simulink model "Snake"  (R2016a)
settings: Solver=VariableStepAuto  StartTime=0.0  StopTime=inf  RelTol=1e-3
libraries: simulink_extras x57, Snake_Lib x44, Arithmetic_Operations_Lib x28, Bit_Multiplexers_Lib x10, Bit_Demultiplexers_Lib x10, commutil2 x6, Decoders_Lib x4, Memory_Blocks_Lib x3, dspsnks4 x1, Miscellaneous x1
(part 1 of 2)
settings Model: Creator=Jozko Mrkvicka  LastModifiedBy=Jozko Mrkvicka

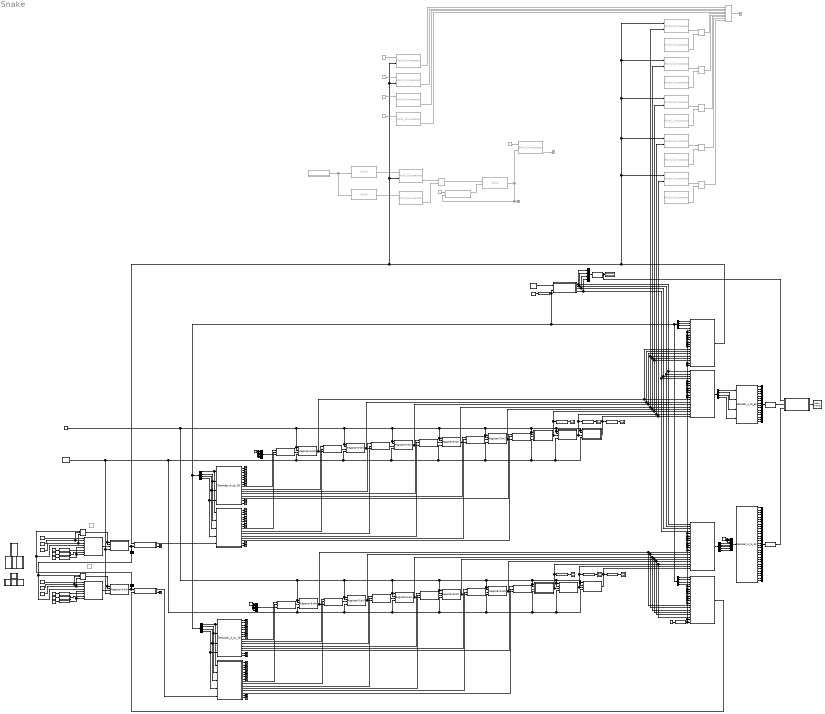
== system Snake ==
  note: New direction is written only when player holds a key.
      | Otherwise old direction keeps latched.
  note: Head is never set to snake position 0 or 1,
  note: TODO:
      |  Add a check to prevent snake from reverting direction. Snake can only turn!!
      | Or figure out how to revert it (idea: maybe it would be possible to shift snake tail directly to it`s head).
  Adder : Subsystem
  Adder1 : Subsystem
  Adder2 : Arithmetic_Operations_Lib/Arithmetic_Operations_Lib/Word_Adder  Commented=on
  Bit to Integer Converter1 : commutil2/Bit to Integer Converter  nbits=32  bitOrder=MSB first  signedOutputValues=Unsigned  outDtype=uint32  outDtypeSigned=Inherit via internal rule
  Bit to Integer Converter2 : commutil2/Bit to Integer Converter  nbits=16  bitOrder=MSB first  signedOutputValues=Unsigned  outDtype=uint32  outDtypeSigned=Inherit via internal rule
  Bit to Integer Converter3 : commutil2/Bit to Integer Converter  nbits=4  bitOrder=MSB first  signedOutputValues=Unsigned  outDtype=uint32  outDtypeSigned=Inherit via internal rule
  Bottom wall : Constant  Commented=on  Value=-1  OutDataTypeStr=boolean
  Bus Creator1 : BusCreator  Inputs=5
  Bus Creator2 : BusCreator  Inputs=5
  Bus Selector : BusSelector  OutputSignals=signal1,signal2,signal3,signal4,signal5
  Bus Selector1 : BusSelector  OutputSignals=signal2,signal3,signal4,signal5
  Bus Selector15 : BusSelector  OutputSignals=signal5
  Bus Selector2 : BusSelector  OutputSignals=signal13,signal14,signal15,signal16
  Bus Selector3 : BusSelector  OutputSignals=signal13,signal14,signal15,signal16
  Bus Selector4 : BusSelector  OutputSignals=signal5
  BusScope(5-bit){,1..5} (6 alike) : Snake_Lib/BusScope(5-bit)
  Counter_4bit : Subsystem
  Decoder_4_to_1 : Decoders_Lib/Decoders_Lib/Decoder_4_to_16
  Decoder_4_to_16 : Decoders_Lib/Decoders_Lib/Decoder_4_to_16
  Decoder_4_to_2 : Decoders_Lib/Decoders_Lib/Decoder_4_to_16
  Decoder_5_to_32 : Decoders_Lib/Decoders_Lib/Decoder_5_to_32
  Delay : Delay  Commented=on  DelayLength=1  InitialCondition=0
  Delay1 : Delay  Commented=on  DelayLength=1  InitialCondition=0
  Demultiplexer_1_to_16(5-bit) : Subsystem  AncestorBlock=Snake_Lib/Demultiplexer_1_to_16(5-bit)
  Demultiplexer_1_to_16(5-bit)1 : Subsystem  AncestorBlock=Snake_Lib/Demultiplexer_1_to_16(5-bit)
  Display{,1..6} (7 alike) : Display
  DisplayClock : simulink_extras/Flip Flops/Clock  period=1
  Down : Constant  Value=0  OutDataTypeStr=boolean
  Game over : Logic  Commented=on  Operator=OR  Inputs=9  IconShape=distinctive  AllPortsSameDT=off  OutDataTypeStr=boolean
  Game over :-( : Terminator  Commented=on
  GameClock : simulink_extras/Flip Flops/Clock  period=6
  General_Purpose_Register_16 (Length of snake) : Memory_Blocks_Lib/Memory_Blocks_Lib/Word  Commented=on
  General_Purpose_Register_16 (Point_to_take(X)) : Memory_Blocks_Lib/Memory_Blocks_Lib/Word  Commented=on
  General_Purpose_Register_16 (Point_to_take(Y)) : Memory_Blocks_Lib/Memory_Blocks_Lib/Word  Commented=on
  Instruction_CMP (Check if snake hit a wall){,,,} (4 alike) : Arithmetic_Operations_Lib/Arithmetic_Operations_Lib/Word_Comparator  Commented=on
  Instruction_CMP (Compare that snake`s head reached new point to take) : Arithmetic_Operations_Lib/Arithmetic_Operations_Lib/Word_Comparator  Commented=on
  Instruction_CMP (Compare that snake`s head reached new point to take) : Arithmetic_Operations_Lib/Arithmetic_Operations_Lib/Word_Comparator  Commented=on
  Instruction_CMP (Check if snake has hit himself){,,1,1..2,2..3,3..4,4} (10 alike) : Arithmetic_Operations_Lib/Arithmetic_Operations_Lib/Word_Comparator  Commented=on
  Instruction_CMP (Check if snake has reached maximal length) : Arithmetic_Operations_Lib/Arithmetic_Operations_Lib/Word_Comparator  Commented=on
  Left : Constant  Value=0  OutDataTypeStr=boolean
  Left wall : Constant  Commented=on  Value=-1  OutDataTypeStr=boolean
  Linear_Feedback_Shift_Register_15bit (random number generator) : Subsystem  Commented=on
  Logical Operator{1..5,9} (6 alike) : Logic  Commented=on  IconShape=distinctive  AllPortsSameDT=off  OutDataTypeStr=boolean
  Logical Operator6 : Logic  Operator=OR  Inputs=3  IconShape=distinctive  AllPortsSameDT=off  OutDataTypeStr=boolean
  Logical Operator7 : Logic  Operator=OR  Inputs=3  IconShape=distinctive  AllPortsSameDT=off  OutDataTypeStr=boolean
  MATLAB Function : MATLAB Function  TreatAsAtomicUnit=on
  Matrix Viewer1 : dspsnks4/Matrix Viewer  ImageParams=off  CMapStr=[0 0.3 0; 0 1 0]  AxisColorbar=on  AxisParams=off  AxisOrigin=Upper left corner  AxisTickMode=Auto  XTickRange=[0 1]  YTickRange=[0 1]  XLabel=X-axis  YLabel=Y-axis  ZLabel=Z-axis  FigPos=[1761 809 160 240]  AxisZoom=on
      settings: YMin=0  YMax=1
  Max length : Constant  Commented=on  Value=16  OutDataTypeStr=boolean
  Multiplexer_2_to_1(5-bit){,1..11} (12 alike) : Snake_Lib/Multiplexer_2_to_1(5-bit)
  Multiplexer_4_to_1_DirSel(5-bit) : Snake_Lib/Multiplexer_4_to_1_DirSel(5-bit)
  Multiplexer_4_to_1_DirSel(5-bit)1 : Snake_Lib/Multiplexer_4_to_1_DirSel(5-bit)
  Mux : Mux  Inputs=16
  Mux1 : Mux  Inputs=32
  Mux2 : Mux  Inputs=8
  Mux3 : Mux
  None1 : Constant  Value=0  OutDataTypeStr=boolean
  None3 : Constant  Value=0  OutDataTypeStr=boolean
  Push Button : Subsystem  DialogController=hmiCreateDDGDialog  IsWebBlock=on  mask(MWDashboardBlock){webBlockId=56926f07-5c30-4489-8789-9949c718d414, webBlockType=pushbutton, ShowInLibBrwoser=on, ShowInitialText=on, HMISrcModelName=Snake}
      mask prompts: webBlockId "WebBlock Id"; webBlockType "WebBlock Type"; HMISrcModelName "Source Model"
      mask Help: helpview([docroot '/mapfiles/simulink.map'], 'hmi_push_button')
      mask Display:
      | model = bdroot(gcb);
      | if strcmp(get_param(model,'BlockDiagramType'), 'library')
      |     image([(matlabroot) '/toolbox/simulink/hmi/icons/PushButton.png']);
      | end
  Push Button1 : Subsystem  DialogController=hmiCreateDDGDialog  IsWebBlock=on  mask(MWDashboardBlock){webBlockId=75882201-b457-4fd9-b9c2-035fbf608d85, webBlockType=pushbutton, ShowInLibBrwoser=on, ShowInitialText=on, HMISrcModelName=Snake}
      mask prompts: webBlockId "WebBlock Id"; webBlockType "WebBlock Type"; HMISrcModelName "Source Model"
      mask Help: helpview([docroot '/mapfiles/simulink.map'], 'hmi_push_button')
      mask Display:
      | model = bdroot(gcb);
      | if strcmp(get_param(model,'BlockDiagramType'), 'library')
      |     image([(matlabroot) '/toolbox/simulink/hmi/icons/PushButton.png']);
      | end
  Push Button2 : Subsystem  DialogController=hmiCreateDDGDialog  IsWebBlock=on  mask(MWDashboardBlock){webBlockId=5ce12bab-ed7e-4f72-890a-6ff3196eb95e, webBlockType=pushbutton, ShowInLibBrwoser=on, ShowInitialText=on, HMISrcModelName=Snake}
      mask prompts: webBlockId "WebBlock Id"; webBlockType "WebBlock Type"; HMISrcModelName "Source Model"
      mask Help: helpview([docroot '/mapfiles/simulink.map'], 'hmi_push_button')
      mask Display:
      | model = bdroot(gcb);
      | if strcmp(get_param(model,'BlockDiagramType'), 'library')
      |     image([(matlabroot) '/toolbox/simulink/hmi/icons/PushButton.png']);
      | end
  Push Button3 : Subsystem  DialogController=hmiCreateDDGDialog  IsWebBlock=on  mask(MWDashboardBlock){webBlockId=28c09741-da14-4d8c-8d5e-be08630d781a, webBlockType=pushbutton, ShowInLibBrwoser=on, ShowInitialText=on, HMISrcModelName=Snake}
      mask prompts: webBlockId "WebBlock Id"; webBlockType "WebBlock Type"; HMISrcModelName "Source Model"
      mask Help: helpview([docroot '/mapfiles/simulink.map'], 'hmi_push_button')
      mask Display:
      | model = bdroot(gcb);
      | if strcmp(get_param(model,'BlockDiagramType'), 'library')
      |     image([(matlabroot) '/toolbox/simulink/hmi/icons/PushButton.png']);
      | end
  Right : Constant  OutDataTypeStr=boolean
  Right wall : Constant  Commented=on  Value=24  OutDataTypeStr=boolean
  Select_Snake_Head(X) : Snake_Lib/Multiplexer_16_to_1(5-bit)
      link override Bus Selector7: OutputSignals=signal1,signal2,signal3,signal4,signal5
  Select_Snake_Head(Y) : Snake_Lib/Multiplexer_16_to_1(5-bit)
      link override Bus Selector7: OutputSignals=signal1,signal2,signal3,signal4,signal5
  Snake Head Position (X) : BusSelector  OutputSignals=signal13,signal14,signal15,signal16
  Snake Head Position (Y) : BusSelector  OutputSignals=signal13,signal14,signal15,signal16
  Snake_X : Snake_Lib/Multiplexer_16_to_1(5-bit)
      link override Bus Selector7: OutputSignals=signal1,signal2,signal3,signal4,signal5
  Snake_X0 : Subsystem
  Snake_X1 : Subsystem
  Snake_X2 : Subsystem
  Snake_X{3..7} (5 alike) : Snake_Lib/Register(5-bit)
  Snake_Y : Snake_Lib/Multiplexer_16_to_1(5-bit)
      link override Bus Creator1: Inputs=5
  Snake_Y0 : Subsystem
  Snake_Y1 : Subsystem
  Snake_Y2 : Subsystem
  Snake_Y{3..7} (5 alike) : Snake_Lib/Register(5-bit)
  Terminator : Terminator  Commented=on
  Terminator{1..3,5..12,20..38,40..51} (42 alike) : Terminator
  Toggle Switch : Subsystem  DialogController=hmiCreateDDGDialog  IsWebBlock=on  mask(MWDashboardBlock){webBlockId=54927be4-b863-4cd1-a632-014d1949c9b6, webBlockType=toggleswitch, ShowInLibBrowser=on, ShowInitialText=on, HMISrcModelName=Snake}
      mask prompts: webBlockId "WebBlock Id"; webBlockType "WebBlock Type"; HMISrcModelName "Source Model"
      mask Help: helpview([docroot '/mapfiles/simulink.map'], 'hmi_toggle_switch')
      mask Display:
      | if strcmp(get_param(bdroot(gcb),'BlockDiagramType'), 'library')
      |     image([(matlabroot) '/toolbox/simulink/hmi/icons/ToggleSwitch.png']);
      | end
  Toggle Switch1 : Subsystem  DialogController=hmiCreateDDGDialog  IsWebBlock=on  mask(MWDashboardBlock){webBlockId=3e42cfe8-21e1-4190-88ba-1de34cedee39, webBlockType=toggleswitch, ShowInLibBrowser=on, ShowInitialText=on, HMISrcModelName=Snake}
      mask prompts: webBlockId "WebBlock Id"; webBlockType "WebBlock Type"; HMISrcModelName "Source Model"
      mask Help: helpview([docroot '/mapfiles/simulink.map'], 'hmi_toggle_switch')
      mask Display:
      | if strcmp(get_param(bdroot(gcb),'BlockDiagramType'), 'library')
      |     image([(matlabroot) '/toolbox/simulink/hmi/icons/ToggleSwitch.png']);
      | end
  Toggle Switch2 : Subsystem  DialogController=hmiCreateDDGDialog  IsWebBlock=on  mask(MWDashboardBlock){webBlockId=c61dffc0-3ed1-4f53-9cab-e3b11f3a47d7, webBlockType=toggleswitch, ShowInLibBrowser=on, ShowInitialText=on, HMISrcModelName=Snake}
      mask prompts: webBlockId "WebBlock Id"; webBlockType "WebBlock Type"; HMISrcModelName "Source Model"
      mask Help: helpview([docroot '/mapfiles/simulink.map'], 'hmi_toggle_switch')
      mask Display:
      | if strcmp(get_param(bdroot(gcb),'BlockDiagramType'), 'library')
      |     image([(matlabroot) '/toolbox/simulink/hmi/icons/ToggleSwitch.png']);
      | end
  Toggle Switch3 : Subsystem  DialogController=hmiCreateDDGDialog  IsWebBlock=on  mask(MWDashboardBlock){webBlockId=f29dcd5f-f5a7-4438-a1c1-2f4b185334c4, webBlockType=toggleswitch, ShowInLibBrowser=on, ShowInitialText=on, HMISrcModelName=Snake}
      mask prompts: webBlockId "WebBlock Id"; webBlockType "WebBlock Type"; HMISrcModelName "Source Model"
      mask Help: helpview([docroot '/mapfiles/simulink.map'], 'hmi_toggle_switch')
      mask Display:
      | if strcmp(get_param(bdroot(gcb),'BlockDiagramType'), 'library')
      |     image([(matlabroot) '/toolbox/simulink/hmi/icons/ToggleSwitch.png']);
      | end
  Top wall : Constant  Commented=on  Value=32  OutDataTypeStr=boolean
  Up : Constant  Value=0  OutDataTypeStr=boolean
  Up1 : Constant  Value=+1  OutDataTypeStr=uint32
  Up2 : Constant  Value=-1  OutDataTypeStr=int8
  Up3 : Constant  Commented=on  Value=+1  OutDataTypeStr=boolean
  Up4 : Constant  Value=+1  OutDataTypeStr=uint32
  Up5 : Constant  Value=-1  OutDataTypeStr=int8
  Up6 : Constant  Value=0  OutDataTypeStr=uint32
  Up7 : Constant  Value=0  OutDataTypeStr=uint32
  Victory!! : Terminator  Commented=on
  X-direction of snake : Subsystem
  Y-direction of snake : Snake_Lib/Register(5-bit)
  const2 : Constant  Value=2  OutDataTypeStr=uint16
  const3 : Constant  OutDataTypeStr=boolean
  const4 : Constant  Value=0  OutDataTypeStr=boolean
  const7 : Constant  Value=0  OutDataTypeStr=boolean
  const8 : Constant  Value=0  OutDataTypeStr=uint8
  const9 : Constant  Value=0  OutDataTypeStr=boolean
  uint_to_bus : Miscellaneous/uint_to_bus
  uint_to_bus(byte){,2..3,5,17} (5 alike) : Snake_Lib/uint_to_bus(byte)
  uint_to_bus(byte)1 : Subsystem
  uint_to_bus(byte)4 : Subsystem
  wires:
  DisplayClock/1 -> Counter_4bit/1(Clock)
  Select_Snake_Head(X)/1 -> Adder/1(Data_In_A(5b)), Instruction_CMP (Check if snake hit a wall)/2, Instruction_CMP (Check if snake hit a wall)/2, Instruction_CMP (Compare that snake`s head reached new point to take)/2, Instruction_CMP (Check if snake has hit himself)4/1, Instruction_CMP (Check if snake has hit himself)3/1, Instruction_CMP (Check if snake has hit himself)2/1, Instruction_CMP (Check if snake has hit himself)1/1, Instruction_CMP (Check if snake has hit himself)/1
  Counter_4bit/2(Addr_2(1b)) -> Mux3/2, Snake_X/2, Snake_Y/2
  Counter_4bit/1(Addr_3(1b)) -> Mux3/1, Snake_X/1, Snake_Y/1
  Counter_4bit/4(Addr_0(1b)) -> Mux3/4, Snake_X/4, Snake_Y/4
  Counter_4bit/3(Addr_1(1b)) -> Mux3/3, Snake_X/3, Snake_Y/3
  Bus Selector1/1 -> Decoder_4_to_16/1  "<signal2>"
  Snake_Y/1 -> Bus Selector/1
  uint_to_bus(byte)/1 -> Multiplexer_4_to_1_DirSel(5-bit)/6
  Multiplexer_4_to_1_DirSel(5-bit)/1 -> X-direction of snake/3(Data(5b))
  uint_to_bus(byte)1/1(Out(5b)) -> Multiplexer_4_to_1_DirSel(5-bit)/7
  Right/1 -> Logical Operator6/2, Multiplexer_4_to_1_DirSel(5-bit)/2
  Left/1 -> Logical Operator6/3, Multiplexer_4_to_1_DirSel(5-bit)/3
  General_Purpose_Register_16 (Point_to_take(X))/1 -> Instruction_CMP (Compare that snake`s head reached new point to take)/1
  Linear_Feedback_Shift_Register_15bit (random number generator)/1(Random_Number(2B)) -> General_Purpose_Register_16 (Point_to_take(Y))/3, General_Purpose_Register_16 (Point_to_take(X))/3
  General_Purpose_Register_16 (Length of snake)/1 -> Terminator/1, Adder2/2, Instruction_CMP (Check if snake has reached maximal length)/2
  Up3/1 -> Adder2/1
  Instruction_CMP (Compare that snake`s head reached new point to take)/5 -> Logical Operator9/1
  Logical Operator9/1 -> General_Purpose_Register_16 (Length of snake)/2
  General_Purpose_Register_16 (Point_to_take(Y))/1 -> Instruction_CMP (Compare that snake`s head reached new point to take)/1
  Instruction_CMP (Compare that snake`s head reached new point to take)/5 -> Logical Operator9/2
  Adder2/1 -> General_Purpose_Register_16 (Length of snake)/3
  Left wall/1 -> Instruction_CMP (Check if snake hit a wall)/1
  Instruction_CMP (Check if snake hit a wall)/5 -> Game over/2
  Right wall/1 -> Instruction_CMP (Check if snake hit a wall)/1
  Instruction_CMP (Check if snake hit a wall)/5 -> Game over/1
  Bottom wall/1 -> Instruction_CMP (Check if snake hit a wall)/1
  Top wall/1 -> Instruction_CMP (Check if snake hit a wall)/1
  Instruction_CMP (Check if snake hit a wall)/5 -> Game over/4
  Instruction_CMP (Check if snake hit a wall)/5 -> Game over/3
  Max length/1 -> Instruction_CMP (Check if snake has reached maximal length)/1
  Instruction_CMP (Check if snake has reached maximal length)/5 -> Victory!!/1
  Game over/1 -> Game over :-(/1
  Instruction_CMP (Check if snake has hit himself)/5 -> Logical Operator1/1
  Instruction_CMP (Check if snake has hit himself)/5 -> Logical Operator1/2
  Logical Operator1/1 -> Game over/5
  Instruction_CMP (Check if snake has hit himself)1/5 -> Logical Operator2/1
  Instruction_CMP (Check if snake has hit himself)1/5 -> Logical Operator2/2
  Instruction_CMP (Check if snake has hit himself)2/5 -> Logical Operator3/1
  Instruction_CMP (Check if snake has hit himself)2/5 -> Logical Operator3/2
  Instruction_CMP (Check if snake has hit himself)3/5 -> Logical Operator4/1
  Instruction_CMP (Check if snake has hit himself)3/5 -> Logical Operator4/2
  Instruction_CMP (Check if snake has hit himself)4/5 -> Logical Operator5/1
  Instruction_CMP (Check if snake has hit himself)4/5 -> Logical Operator5/2
  Logical Operator2/1 -> Game over/6
  Logical Operator3/1 -> Game over/7
  Logical Operator4/1 -> Game over/8
  Logical Operator5/1 -> Game over/9
  Decoder_4_to_16/1 -> Mux/1
  Decoder_4_to_16/2 -> Mux/2
  Decoder_4_to_16/3 -> Mux/3
  Decoder_4_to_16/4 -> Mux/4
  Decoder_4_to_16/5 -> Mux/5
  Decoder_4_to_16/6 -> Mux/6
  Decoder_4_to_16/7 -> Mux/7
  Decoder_4_to_16/8 -> Mux/8
  Decoder_4_to_16/9 -> Mux/9
  Decoder_4_to_16/10 -> Mux/10
  Decoder_4_to_16/11 -> Mux/11
  Decoder_4_to_16/12 -> Mux/12
  Decoder_4_to_16/13 -> Mux/13
  Decoder_4_to_16/14 -> Mux/14
  Decoder_4_to_16/15 -> Mux/15
  Decoder_4_to_16/16 -> Mux/16
  Mux/1 -> Bit to Integer Converter2/1
  Bus Selector1/2 -> Decoder_4_to_16/2  "<signal3>"
  Bus Selector1/3 -> Decoder_4_to_16/3  "<signal4>"
  Bus Selector1/4 -> Decoder_4_to_16/4  "<signal5>"
  Decoder_5_to_32/1 -> Mux1/1
  Decoder_5_to_32/2 -> Mux1/2
  Decoder_5_to_32/3 -> Mux1/3
  Decoder_5_to_32/4 -> Mux1/4
  Decoder_5_to_32/5 -> Mux1/5
  Decoder_5_to_32/6 -> Mux1/6
  Decoder_5_to_32/7 -> Mux1/7
  Decoder_5_to_32/8 -> Mux1/8
  Decoder_5_to_32/9 -> Mux1/9
  Decoder_5_to_32/10 -> Mux1/10
  Decoder_5_to_32/11 -> Mux1/11
  Decoder_5_to_32/12 -> Mux1/12
  Decoder_5_to_32/13 -> Mux1/13
  Decoder_5_to_32/14 -> Mux1/14
  Decoder_5_to_32/15 -> Mux1/15
  Decoder_5_to_32/16 -> Mux1/16
  Decoder_5_to_32/17 -> Mux1/17
  Decoder_5_to_32/18 -> Mux1/18
  Decoder_5_to_32/19 -> Mux1/19
  Decoder_5_to_32/20 -> Mux1/20
  Decoder_5_to_32/21 -> Mux1/21
  Decoder_5_to_32/22 -> Mux1/22
  Decoder_5_to_32/23 -> Mux1/23
  Decoder_5_to_32/24 -> Mux1/24
  Decoder_5_to_32/25 -> Mux1/25
  Decoder_5_to_32/26 -> Mux1/26
  Decoder_5_to_32/27 -> Mux1/27
  Decoder_5_to_32/28 -> Mux1/28
  Decoder_5_to_32/29 -> Mux1/29
  Decoder_5_to_32/30 -> Mux1/30
  Decoder_5_to_32/31 -> Mux1/31
  Mux1/1 -> Bit to Integer Converter1/1
  Decoder_5_to_32/32 -> Mux1/32
  const2/1 -> uint_to_bus/1
  Bus Selector/1 -> Mux2/4  "<signal1>"
  Bus Selector/2 -> Mux2/5  "<signal2>"
  Bus Selector/3 -> Mux2/6  "<signal3>"
  Bus Selector/4 -> Mux2/7  "<signal4>"
  Bus Selector/5 -> Mux2/8  "<signal5>"
  Mux2/1 -> Decoder_5_to_32/1
  const7/1 -> Mux2/2, Mux2/3, Mux2/1
  Snake_X/1 -> Bus Selector1/1
  const9/1 -> Bus Creator1/5, Bus Creator1/4, Bus Creator1/3, Bus Creator1/2, Bus Creator1/1
  Bus Creator1/1 -> Multiplexer_2_to_1(5-bit)/3
  Mux3/1 -> Bit to Integer Converter3/1
  Adder/2(Carry_Out(1b)) -> Terminator1/1
  Adder/1(Data_Out(5b)) -> Demultiplexer_1_to_16(5-bit)/5(Data(5b))
  MATLAB Function/1(Framebuffer) -> Matrix Viewer1/1
  Bit to Integer Converter2/1 -> MATLAB Function/2(x)
  Bit to Integer Converter1/1 -> MATLAB Function/3(y)
  Snake_X7/1 -> Multiplexer_2_to_1(5-bit)1/3, Snake_X/13, Select_Snake_Head(X)/13
  Snake_X6/1 -> Multiplexer_2_to_1(5-bit)2/3, Snake_X/14, Select_Snake_Head(X)/14
  Snake_X5/1 -> Multiplexer_2_to_1(5-bit)3/3, Snake_X/15, Select_Snake_Head(X)/15
  Snake_X4/1 -> Multiplexer_2_to_1(5-bit)4/3, Instruction_CMP (Check if snake has hit himself)/2, Select_Snake_Head(X)/16, Snake_X/16
  Snake_X3/1 -> Multiplexer_2_to_1(5-bit)5/3, Instruction_CMP (Check if snake has hit himself)1/2, Select_Snake_Head(X)/17, Snake_X/17
  Snake_X2/1(DataOut(5b)) -> Snake_X1/3(Data(5b)), Instruction_CMP (Check if snake has hit himself)2/2, Select_Snake_Head(X)/18, Snake_X/18, BusScope(5-bit)1/1
  Snake_X1/1(DataOut(5b)) -> BusScope(5-bit)/1, Snake_X/19, Instruction_CMP (Check if snake has hit himself)3/2, Snake_X0/3(Data(5b))
  Snake_X0/1(DataOut(5b)) -> BusScope(5-bit)2/1, Snake_X/20, Instruction_CMP (Check if snake has hit himself)4/2
  Bit to Integer Converter3/1 -> MATLAB Function/1(cnt), Display/1
  Bus Selector4/1 -> Multiplexer_4_to_1_DirSel(5-bit)/4, Logical Operator6/1  "<signal5>"
  uint_to_bus(byte)2/1 -> Multiplexer_4_to_1_DirSel(5-bit)/8, Multiplexer_4_to_1_DirSel(5-bit)/5
  None1/1 -> Multiplexer_4_to_1_DirSel(5-bit)/1
  Bus Selector2/1 -> Select_Snake_Head(X)/1  "<signal13>"
  Bus Selector2/2 -> Select_Snake_Head(X)/2  "<signal14>"
  Bus Selector2/3 -> Select_Snake_Head(X)/3  "<signal15>"
  Bus Selector2/4 -> Select_Snake_Head(X)/4  "<signal16>"
  const8/1 -> uint_to_bus(byte)17/1
  Snake Head Position (X)/1 -> Decoder_4_to_1/1, Demultiplexer_1_to_16(5-bit)/1(Addr3(1b))  "<signal13>"
  Snake Head Position (X)/2 -> Decoder_4_to_1/2, Demultiplexer_1_to_16(5-bit)/2(Addr2(1b))  "<signal14>"
  Snake Head Position (X)/3 -> Decoder_4_to_1/3, Demultiplexer_1_to_16(5-bit)/3(Addr1(1b))  "<signal15>"
  Snake Head Position (X)/4 -> Decoder_4_to_1/4, Demultiplexer_1_to_16(5-bit)/4(Addr0(1b))  "<signal16>"
  uint_to_bus/1 -> Counter_4bit/2(Snake_Length(2B)), Bus Selector3/1, Bus Selector2/1, Snake Head Position (Y)/1, Snake Head Position (X)/1
  Demultiplexer_1_to_16(5-bit)/15(Data_01(5b)) -> Terminator2/1
  Demultiplexer_1_to_16(5-bit)/16(Data_00(5b)) -> Terminator3/1
  Multiplexer_2_to_1(5-bit)/1 -> Snake_X7/3
  Multiplexer_2_to_1(5-bit)1/1 -> Snake_X6/3
  Multiplexer_2_to_1(5-bit)2/1 -> Snake_X5/3
  Multiplexer_2_to_1(5-bit)3/1 -> Snake_X4/3
  Multiplexer_2_to_1(5-bit)4/1 -> Snake_X3/3
  Multiplexer_2_to_1(5-bit)5/1 -> Snake_X2/3(Data(5b))
  Decoder_4_to_1/9 -> Multiplexer_2_to_1(5-bit)/1
  Demultiplexer_1_to_16(5-bit)/9(Data_07(5b)) -> Multiplexer_2_to_1(5-bit)/2
  Decoder_4_to_1/10 -> Multiplexer_2_to_1(5-bit)1/1
  Demultiplexer_1_to_16(5-bit)/10(Data_06(5b)) -> Multiplexer_2_to_1(5-bit)1/2
  Decoder_4_to_1/11 -> Multiplexer_2_to_1(5-bit)2/1
  Demultiplexer_1_to_16(5-bit)/11(Data_05(5b)) -> Multiplexer_2_to_1(5-bit)2/2
  Decoder_4_to_1/12 -> Multiplexer_2_to_1(5-bit)3/1
  Demultiplexer_1_to_16(5-bit)/12(Data_04(5b)) -> Multiplexer_2_to_1(5-bit)3/2
  Decoder_4_to_1/13 -> Multiplexer_2_to_1(5-bit)4/1
  Demultiplexer_1_to_16(5-bit)/13(Data_03(5b)) -> Multiplexer_2_to_1(5-bit)4/2
  Decoder_4_to_1/14 -> Multiplexer_2_to_1(5-bit)5/1
  Demultiplexer_1_to_16(5-bit)/14(Data_02(5b)) -> Multiplexer_2_to_1(5-bit)5/2
  Demultiplexer_1_to_16(5-bit)/1(Data_15(5b)) -> Terminator20/1
  Demultiplexer_1_to_16(5-bit)/2(Data_14(5b)) -> Terminator21/1
  Demultiplexer_1_to_16(5-bit)/3(Data_13(5b)) -> Terminator22/1
  Demultiplexer_1_to_16(5-bit)/4(Data_12(5b)) -> Terminator23/1
  Demultiplexer_1_to_16(5-bit)/5(Data_11(5b)) -> Terminator24/1
  Demultiplexer_1_to_16(5-bit)/6(Data_10(5b)) -> Terminator25/1
  Demultiplexer_1_to_16(5-bit)/7(Data_09(5b)) -> Terminator26/1
  Demultiplexer_1_to_16(5-bit)/8(Data_08(5b)) -> Terminator27/1
  Decoder_4_to_1/1 -> Terminator28/1
  Decoder_4_to_1/2 -> Terminator29/1
  Decoder_4_to_1/3 -> Terminator30/1
  Decoder_4_to_1/4 -> Terminator31/1
  Decoder_4_to_1/5 -> Terminator32/1
  Decoder_4_to_1/6 -> Terminator33/1
  Decoder_4_to_1/7 -> Terminator34/1
  Decoder_4_to_1/8 -> Terminator35/1
  Decoder_4_to_1/15 -> Terminator36/1
  Decoder_4_to_1/16 -> Terminator37/1
  Up1/1 -> uint_to_bus(byte)/1
  Up2/1 -> uint_to_bus(byte)1/1(In(5b))
  Up6/1 -> uint_to_bus(byte)2/1
  BusScope(5-bit)/1 -> Display2/1
  BusScope(5-bit)1/1 -> Display1/1
  BusScope(5-bit)2/1 -> Display3/1
  GameClock/1 -> Y-direction of snake/4, X-direction of snake/4(CLK), Snake_X0/4(CLK), Snake_X1/4(CLK), Snake_X2/4(CLK), Snake_X3/4, Snake_X4/4, Snake_X5/4, Snake_X6/4, Snake_X7/4, Snake_Y0/4(CLK), Snake_Y1/4(CLK), Snake_Y2/4(CLK), Snake_Y3/4, Snake_Y4/4, Snake_Y5/4, Snake_Y6/4, Snake_Y7/4
  const4/1 -> Bus Creator2/5, Bus Creator2/4, Bus Creator2/3, Bus Creator2/2, Bus Creator2/1
  Bus Creator2/1 -> Multiplexer_2_to_1(5-bit)6/3
  Snake_Y7/1 -> Multiplexer_2_to_1(5-bit)7/3, Snake_Y/13, Select_Snake_Head(Y)/13
  Snake_Y6/1 -> Multiplexer_2_to_1(5-bit)8/3, Snake_Y/14, Select_Snake_Head(Y)/14
  Snake_Y5/1 -> Multiplexer_2_to_1(5-bit)9/3, Snake_Y/15, Select_Snake_Head(Y)/15
  Snake_Y4/1 -> Multiplexer_2_to_1(5-bit)10/3, Snake_Y/16, Select_Snake_Head(Y)/16
  Snake_Y3/1 -> Multiplexer_2_to_1(5-bit)11/3, Snake_Y/17, Select_Snake_Head(Y)/17
  Snake_Y2/1(DataOut(5b)) -> Snake_Y1/3(Data(5b)), Snake_Y/18, Select_Snake_Head(Y)/18, BusScope(5-bit)4/1
  Snake_Y1/1(DataOut(5b)) -> Snake_Y/19, BusScope(5-bit)3/1, Snake_Y0/3(Data(5b))
  Snake_Y0/1(DataOut(5b)) -> Snake_Y/20, BusScope(5-bit)5/1
  Snake Head Position (Y)/1 -> Decoder_4_to_2/1, Demultiplexer_1_to_16(5-bit)1/1(Addr3(1b))  "<signal13>"
  Snake Head Position (Y)/2 -> Decoder_4_to_2/2, Demultiplexer_1_to_16(5-bit)1/2(Addr2(1b))  "<signal14>"
  Snake Head Position (Y)/3 -> Decoder_4_to_2/3, Demultiplexer_1_to_16(5-bit)1/3(Addr1(1b))  "<signal15>"
  Snake Head Position (Y)/4 -> Decoder_4_to_2/4, Demultiplexer_1_to_16(5-bit)1/4(Addr0(1b))  "<signal16>"
  Demultiplexer_1_to_16(5-bit)1/15(Data_01(5b)) -> Terminator5/1
  Demultiplexer_1_to_16(5-bit)1/16(Data_00(5b)) -> Terminator43/1
  Multiplexer_2_to_1(5-bit)6/1 -> Snake_Y7/3
  Multiplexer_2_to_1(5-bit)7/1 -> Snake_Y6/3
  Multiplexer_2_to_1(5-bit)8/1 -> Snake_Y5/3
  Multiplexer_2_to_1(5-bit)9/1 -> Snake_Y4/3
  Multiplexer_2_to_1(5-bit)10/1 -> Snake_Y3/3
  Multiplexer_2_to_1(5-bit)11/1 -> Snake_Y2/3(Data(5b))
  Decoder_4_to_2/9 -> Multiplexer_2_to_1(5-bit)6/1
  Demultiplexer_1_to_16(5-bit)1/9(Data_07(5b)) -> Multiplexer_2_to_1(5-bit)6/2
  Decoder_4_to_2/10 -> Multiplexer_2_to_1(5-bit)7/1
  Demultiplexer_1_to_16(5-bit)1/10(Data_06(5b)) -> Multiplexer_2_to_1(5-bit)7/2
  Decoder_4_to_2/11 -> Multiplexer_2_to_1(5-bit)8/1
  Demultiplexer_1_to_16(5-bit)1/11(Data_05(5b)) -> Multiplexer_2_to_1(5-bit)8/2
  Decoder_4_to_2/12 -> Multiplexer_2_to_1(5-bit)9/1
  Demultiplexer_1_to_16(5-bit)1/12(Data_04(5b)) -> Multiplexer_2_to_1(5-bit)9/2
  Decoder_4_to_2/13 -> Multiplexer_2_to_1(5-bit)10/1
  Demultiplexer_1_to_16(5-bit)1/13(Data_03(5b)) -> Multiplexer_2_to_1(5-bit)10/2
  Decoder_4_to_2/14 -> Multiplexer_2_to_1(5-bit)11/1
  Demultiplexer_1_to_16(5-bit)1/14(Data_02(5b)) -> Multiplexer_2_to_1(5-bit)11/2
  Demultiplexer_1_to_16(5-bit)1/1(Data_15(5b)) -> Terminator6/1
  Demultiplexer_1_to_16(5-bit)1/2(Data_14(5b)) -> Terminator7/1
  Demultiplexer_1_to_16(5-bit)1/3(Data_13(5b)) -> Terminator8/1
  Demultiplexer_1_to_16(5-bit)1/4(Data_12(5b)) -> Terminator9/1
  Demultiplexer_1_to_16(5-bit)1/5(Data_11(5b)) -> Terminator10/1
  Demultiplexer_1_to_16(5-bit)1/6(Data_10(5b)) -> Terminator11/1
  Demultiplexer_1_to_16(5-bit)1/7(Data_09(5b)) -> Terminator12/1
  Demultiplexer_1_to_16(5-bit)1/8(Data_08(5b)) -> Terminator40/1
  Decoder_4_to_2/1 -> Terminator41/1
  Decoder_4_to_2/2 -> Terminator42/1
  Decoder_4_to_2/3 -> Terminator44/1
  Decoder_4_to_2/4 -> Terminator45/1
  Decoder_4_to_2/5 -> Terminator46/1
  Decoder_4_to_2/6 -> Terminator47/1
  Decoder_4_to_2/7 -> Terminator48/1
  Decoder_4_to_2/8 -> Terminator49/1
  Decoder_4_to_2/15 -> Terminator50/1
  Decoder_4_to_2/16 -> Terminator51/1
  BusScope(5-bit)3/1 -> Display5/1
  BusScope(5-bit)4/1 -> Display4/1
  BusScope(5-bit)5/1 -> Display6/1
  Bus Selector3/1 -> Select_Snake_Head(Y)/1  "<signal13>"
  Bus Selector3/2 -> Select_Snake_Head(Y)/2  "<signal14>"
  Bus Selector3/3 -> Select_Snake_Head(Y)/3  "<signal15>"
  Bus Selector3/4 -> Select_Snake_Head(Y)/4  "<signal16>"
  uint_to_bus(byte)17/1 -> Select_Snake_Head(X)/5, Select_Snake_Head(X)/6, Select_Snake_Head(X)/7, Select_Snake_Head(X)/8, Select_Snake_Head(X)/9, Select_Snake_Head(X)/10, Select_Snake_Head(X)/11, Select_Snake_Head(X)/12, Select_Snake_Head(X)/19, Select_Snake_Head(X)/20, Snake_X/5, Snake_X/6, Snake_X/7, Snake_X/8, Snake_X/9, Snake_X/10, Snake_X/11, Snake_X/12, Snake_Y/5, Snake_Y/6, Snake_Y/7, Snake_Y/8, Snake_Y/9, Snake_Y/10, Snake_Y/11, Snake_Y/12, Select_Snake_Head(Y)/5, Select_Snake_Head(Y)/6, Select_Snake_Head(Y)/7, Select_Snake_Head(Y)/8, Select_Snake_Head(Y)/9, Select_Snake_Head(Y)/10, Select_Snake_Head(Y)/11, Select_Snake_Head(Y)/12, Select_Snake_Head(Y)/19, Select_Snake_Head(Y)/20
  uint_to_bus(byte)3/1 -> Multiplexer_4_to_1_DirSel(5-bit)1/6
  Multiplexer_4_to_1_DirSel(5-bit)1/1 -> Y-direction of snake/3
  uint_to_bus(byte)4/1(Out(5b)) -> Multiplexer_4_to_1_DirSel(5-bit)1/7
  Down/1 -> Logical Operator7/2, Multiplexer_4_to_1_DirSel(5-bit)1/2
  Up/1 -> Logical Operator7/3, Multiplexer_4_to_1_DirSel(5-bit)1/3
  Adder1/2(Carry_Out(1b)) -> Terminator38/1
  uint_to_bus(byte)5/1 -> Multiplexer_4_to_1_DirSel(5-bit)1/8, Multiplexer_4_to_1_DirSel(5-bit)1/5
  None3/1 -> Multiplexer_4_to_1_DirSel(5-bit)1/1
  Up4/1 -> uint_to_bus(byte)3/1
  Up5/1 -> uint_to_bus(byte)4/1(In(5b))
  Up7/1 -> uint_to_bus(byte)5/1
  Adder1/1(Data_Out(5b)) -> Demultiplexer_1_to_16(5-bit)1/5(Data(5b))
  Select_Snake_Head(Y)/1 -> Adder1/2(Data_In_B(5b))
  X-direction of snake/1(DataOut(5b)) -> Bus Selector15/1, Adder/2(Data_In_B(5b))
  Y-direction of snake/1 -> Adder1/1(Data_In_A(5b)), Bus Selector4/1
  const3/1 -> Snake_Y0/2(Write(1b)), Snake_Y0/1(Select(1b)), Snake_Y1/1(Select(1b)), Snake_Y1/2(Write(1b)), Snake_Y2/1(Select(1b)), Snake_Y2/2(Write(1b)), Snake_Y3/2, Snake_Y3/1, Snake_Y4/1, Snake_Y4/2, Snake_Y5/1, Snake_Y5/2, Snake_Y6/1, Snake_Y6/2, Snake_Y7/1, Snake_Y7/2, Snake_X0/2(Write(1b)), Snake_X0/1(Select(1b)), Snake_X1/2(Write(1b)), Snake_X1/1(Select(1b)), Snake_X2/1(Select(1b)), Snake_X2/2(Write(1b)), Snake_X3/1, Snake_X3/2, Snake_X4/2, Snake_X4/1, Snake_X5/2, Snake_X5/1, Snake_X6/1, Snake_X6/2, Snake_X7/2, Snake_X7/1
  Logical Operator6/1 -> X-direction of snake/1(Select(1b)), X-direction of snake/2(Write(1b))
  Logical Operator7/1 -> Y-direction of snake/1, Y-direction of snake/2
  Bus Selector15/1 -> Logical Operator7/1, Multiplexer_4_to_1_DirSel(5-bit)1/4  "<signal5>"

== system Snake/Adder ==
  Data_In_A(5b) : Inport
  Data_In_B(5b) : Inport  Port=2
  Bit_Adder_(0) : Arithmetic_Operations_Lib/Arithmetic_Operations_Lib/Bit_Adder
  Bit_Adder_(1) : Arithmetic_Operations_Lib/Arithmetic_Operations_Lib/Bit_Adder
  Bit_Adder_(2) : Arithmetic_Operations_Lib/Arithmetic_Operations_Lib/Bit_Adder
  Bit_Adder_(3) : Arithmetic_Operations_Lib/Arithmetic_Operations_Lib/Bit_Adder
  Bit_Adder_(4) : Arithmetic_Operations_Lib/Arithmetic_Operations_Lib/Bit_Adder
  Bus Creator : BusCreator  Inputs=5
  Bus Selector : BusSelector  OutputSignals=signal1,signal2,signal3,signal4,signal5
  Bus Selector1 : BusSelector  OutputSignals=signal1,signal2,signal3,signal4,signal5
  Constant : Constant  Value=0
  Data_Out(5b) : Outport
  Carry_Out(1b) : Outport  Port=2
  wires:
  Bit_Adder_(4)/2 -> Carry_Out(1b)/1
  Data_In_A(5b)/1 -> Bus Selector/1
  Data_In_B(5b)/1 -> Bus Selector1/1
  Bus Creator/1 -> Data_Out(5b)/1
  Bit_Adder_(0)/1 -> Bus Creator/5
  Bit_Adder_(1)/1 -> Bus Creator/4
  Bit_Adder_(2)/1 -> Bus Creator/3
  Bit_Adder_(4)/1 -> Bus Creator/1
  Bit_Adder_(3)/1 -> Bus Creator/2
  Bus Selector/1 -> Bit_Adder_(4)/1  "<signal1>"
  Bus Selector/2 -> Bit_Adder_(3)/1  "<signal2>"
  Bus Selector/3 -> Bit_Adder_(2)/1  "<signal3>"
  Bus Selector/4 -> Bit_Adder_(1)/1  "<signal4>"
  Bus Selector/5 -> Bit_Adder_(0)/1  "<signal5>"
  Bus Selector1/1 -> Bit_Adder_(4)/2  "<signal1>"
  Bus Selector1/2 -> Bit_Adder_(3)/2  "<signal2>"
  Bus Selector1/3 -> Bit_Adder_(2)/2  "<signal3>"
  Bus Selector1/4 -> Bit_Adder_(1)/2  "<signal4>"
  Bus Selector1/5 -> Bit_Adder_(0)/2  "<signal5>"
  Constant/1 -> Bit_Adder_(0)/3
  Bit_Adder_(0)/2 -> Bit_Adder_(1)/3
  Bit_Adder_(1)/2 -> Bit_Adder_(2)/3
  Bit_Adder_(2)/2 -> Bit_Adder_(3)/3
  Bit_Adder_(3)/2 -> Bit_Adder_(4)/3

== system Snake/Adder1 ==
  Data_In_A(5b) : Inport
  Data_In_B(5b) : Inport  Port=2
  Bit_Adder_(0) : Arithmetic_Operations_Lib/Arithmetic_Operations_Lib/Bit_Adder
  Bit_Adder_(1) : Arithmetic_Operations_Lib/Arithmetic_Operations_Lib/Bit_Adder
  Bit_Adder_(2) : Arithmetic_Operations_Lib/Arithmetic_Operations_Lib/Bit_Adder
  Bit_Adder_(3) : Arithmetic_Operations_Lib/Arithmetic_Operations_Lib/Bit_Adder
  Bit_Adder_(4) : Arithmetic_Operations_Lib/Arithmetic_Operations_Lib/Bit_Adder
  Bus Creator : BusCreator  Inputs=5
  Bus Selector : BusSelector  OutputSignals=signal1,signal2,signal3,signal4,signal5
  Bus Selector1 : BusSelector  OutputSignals=signal1,signal2,signal3,signal4,signal5
  Constant : Constant  Value=0
  Data_Out(5b) : Outport
  Carry_Out(1b) : Outport  Port=2
  wires:
  Bit_Adder_(4)/2 -> Carry_Out(1b)/1
  Data_In_A(5b)/1 -> Bus Selector/1
  Data_In_B(5b)/1 -> Bus Selector1/1
  Bus Creator/1 -> Data_Out(5b)/1
  Bit_Adder_(0)/1 -> Bus Creator/5
  Bit_Adder_(1)/1 -> Bus Creator/4
  Bit_Adder_(2)/1 -> Bus Creator/3
  Bit_Adder_(4)/1 -> Bus Creator/1
  Bit_Adder_(3)/1 -> Bus Creator/2
  Bus Selector/1 -> Bit_Adder_(4)/1  "<signal1>"
  Bus Selector/2 -> Bit_Adder_(3)/1  "<signal2>"
  Bus Selector/3 -> Bit_Adder_(2)/1  "<signal3>"
  Bus Selector/4 -> Bit_Adder_(1)/1  "<signal4>"
  Bus Selector/5 -> Bit_Adder_(0)/1  "<signal5>"
  Bus Selector1/1 -> Bit_Adder_(4)/2  "<signal1>"
  Bus Selector1/2 -> Bit_Adder_(3)/2  "<signal2>"
  Bus Selector1/3 -> Bit_Adder_(2)/2  "<signal3>"
  Bus Selector1/4 -> Bit_Adder_(1)/2  "<signal4>"
  Bus Selector1/5 -> Bit_Adder_(0)/2  "<signal5>"
  Constant/1 -> Bit_Adder_(0)/3
  Bit_Adder_(0)/2 -> Bit_Adder_(1)/3
  Bit_Adder_(1)/2 -> Bit_Adder_(2)/3
  Bit_Adder_(2)/2 -> Bit_Adder_(3)/3
  Bit_Adder_(3)/2 -> Bit_Adder_(4)/3

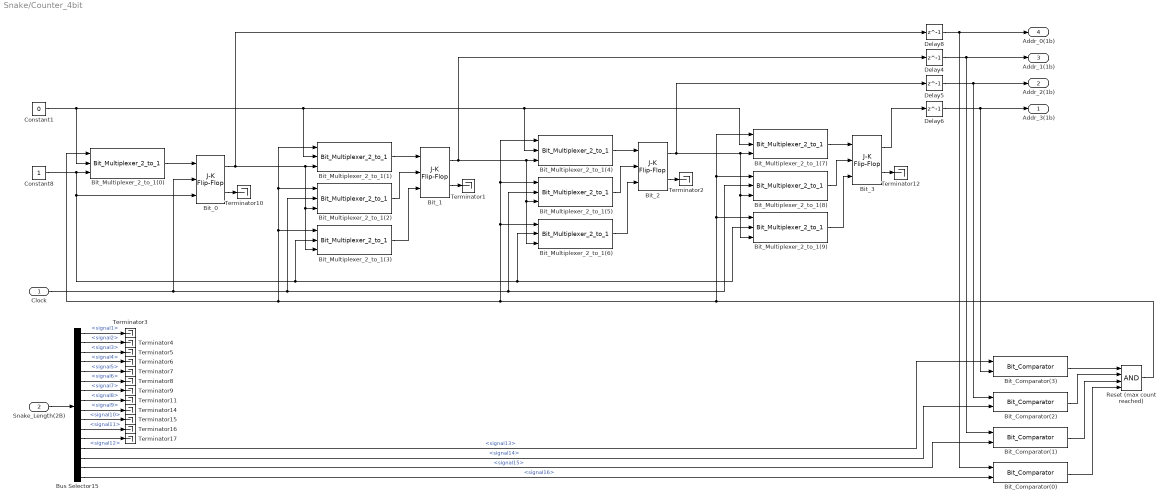
== system Snake/Counter_4bit ==
  Clock : Inport
  Snake_Length(2B) : Inport  Port=2
  Bit_{0..3} (4 alike) : simulink_extras/Flip Flops/J-K Flip-Flop  initial_condition=0
  Bit_Comparator(0) : Snake_Lib/Bit_Comparator
  Bit_Comparator(1) : Snake_Lib/Bit_Comparator
  Bit_Comparator(2) : Snake_Lib/Bit_Comparator
  Bit_Comparator(3) : Snake_Lib/Bit_Comparator
  Bit_Multiplexer_2_to_1(0) : Bit_Multiplexers_Lib/Bit_Multiplexers_Lib/Bit_Multiplexer_2_to_1
  Bit_Multiplexer_2_to_1(1) : Bit_Multiplexers_Lib/Bit_Multiplexers_Lib/Bit_Multiplexer_2_to_1
  Bit_Multiplexer_2_to_1(2) : Bit_Multiplexers_Lib/Bit_Multiplexers_Lib/Bit_Multiplexer_2_to_1
  Bit_Multiplexer_2_to_1(3) : Bit_Multiplexers_Lib/Bit_Multiplexers_Lib/Bit_Multiplexer_2_to_1
  Bit_Multiplexer_2_to_1(4) : Bit_Multiplexers_Lib/Bit_Multiplexers_Lib/Bit_Multiplexer_2_to_1
  Bit_Multiplexer_2_to_1(5) : Bit_Multiplexers_Lib/Bit_Multiplexers_Lib/Bit_Multiplexer_2_to_1
  Bit_Multiplexer_2_to_1(6) : Bit_Multiplexers_Lib/Bit_Multiplexers_Lib/Bit_Multiplexer_2_to_1
  Bit_Multiplexer_2_to_1(7) : Bit_Multiplexers_Lib/Bit_Multiplexers_Lib/Bit_Multiplexer_2_to_1
  Bit_Multiplexer_2_to_1(8) : Bit_Multiplexers_Lib/Bit_Multiplexers_Lib/Bit_Multiplexer_2_to_1
  Bit_Multiplexer_2_to_1(9) : Bit_Multiplexers_Lib/Bit_Multiplexers_Lib/Bit_Multiplexer_2_to_1
  Bus Selector15 : BusSelector  OutputSignals=signal1,signal2,signal3,signal4,signal5,signal6,signal7,signal8,signal9,signal10,signal11,signal12,signal13,signal14,signal15,signal16
  Constant1 : Constant  Value=0  OutDataTypeStr=boolean
  Constant8 : Constant  OutDataTypeStr=boolean
  Delay{4..6,8} (4 alike) : Delay  DelayLength=1  InitialCondition=0
  Reset (max count reached) : Logic  Inputs=4  IconShape=distinctive  AllPortsSameDT=off  OutDataTypeStr=boolean
  Terminator{1..12,14..17} (16 alike) : Terminator
  Addr_3(1b) : Outport
  Addr_2(1b) : Outport  Port=2
  Addr_1(1b) : Outport  Port=3
  Addr_0(1b) : Outport  Port=4
  wires:
  Bit_2/1 -> Delay5/1, Bit_Multiplexer_2_to_1(8)/3, Bit_Multiplexer_2_to_1(9)/3, Bit_Multiplexer_2_to_1(7)/3
  Bit_2/2 -> Terminator2/1
  Bit_1/2 -> Terminator1/1
  Bit_1/1 -> Delay4/1, Bit_Multiplexer_2_to_1(4)/3, Bit_Multiplexer_2_to_1(6)/3, Bit_Multiplexer_2_to_1(5)/3
  Bit_0/1 -> Delay8/1, Bit_Multiplexer_2_to_1(3)/3, Bit_Multiplexer_2_to_1(2)/3, Bit_Multiplexer_2_to_1(1)/3
  Bit_3/1 -> Delay6/1
  Bit_3/2 -> Terminator12/1
  Bit_0/2 -> Terminator10/1
  Snake_Length(2B)/1 -> Bus Selector15/1
  Bus Selector15/1 -> Terminator3/1  "<signal1>"
  Bus Selector15/2 -> Terminator4/1  "<signal2>"
  Bus Selector15/3 -> Terminator5/1  "<signal3>"
  Bus Selector15/4 -> Terminator6/1  "<signal4>"
  Bus Selector15/5 -> Terminator7/1  "<signal5>"
  Bus Selector15/6 -> Terminator8/1  "<signal6>"
  Bus Selector15/7 -> Terminator9/1  "<signal7>"
  Bus Selector15/8 -> Terminator11/1  "<signal8>"
  Bus Selector15/9 -> Terminator14/1  "<signal9>"
  Bus Selector15/10 -> Terminator15/1  "<signal10>"
  Bus Selector15/11 -> Terminator16/1  "<signal11>"
  Bus Selector15/12 -> Terminator17/1  "<signal12>"
  Bus Selector15/16 -> Bit_Comparator(0)/2  "<signal16>"
  Bus Selector15/15 -> Bit_Comparator(1)/2  "<signal15>"
  Bus Selector15/14 -> Bit_Comparator(2)/2  "<signal14>"
  Bus Selector15/13 -> Bit_Comparator(3)/1  "<signal13>"
  Bit_Comparator(3)/1 -> Reset (max count reached)/1
  Bit_Comparator(2)/1 -> Reset (max count reached)/2
  Bit_Comparator(1)/1 -> Reset (max count reached)/3
  Bit_Comparator(0)/1 -> Reset (max count reached)/4
  Bit_Multiplexer_2_to_1(7)/1 -> Bit_3/1
  Bit_Multiplexer_2_to_1(9)/1 -> Bit_3/3
  Bit_Multiplexer_2_to_1(8)/1 -> Bit_3/2
  Reset (max count reached)/1 -> Bit_Multiplexer_2_to_1(0)/1, Bit_Multiplexer_2_to_1(3)/1, Bit_Multiplexer_2_to_1(2)/1, Bit_Multiplexer_2_to_1(1)/1, Bit_Multiplexer_2_to_1(4)/1, Bit_Multiplexer_2_to_1(5)/1, Bit_Multiplexer_2_to_1(6)/1, Bit_Multiplexer_2_to_1(7)/1, Bit_Multiplexer_2_to_1(8)/1, Bit_Multiplexer_2_to_1(9)/1
  Constant1/1 -> Bit_Multiplexer_2_to_1(0)/2, Bit_Multiplexer_2_to_1(1)/2, Bit_Multiplexer_2_to_1(4)/2, Bit_Multiplexer_2_to_1(7)/2
  Constant8/1 -> Bit_Multiplexer_2_to_1(3)/2, Bit_Multiplexer_2_to_1(9)/2, Bit_Multiplexer_2_to_1(6)/2, Bit_0/3, Bit_Multiplexer_2_to_1(0)/3
  Bit_Multiplexer_2_to_1(4)/1 -> Bit_2/1
  Bit_Multiplexer_2_to_1(5)/1 -> Bit_2/2
  Bit_Multiplexer_2_to_1(6)/1 -> Bit_2/3
  Bit_Multiplexer_2_to_1(1)/1 -> Bit_1/1
  Bit_Multiplexer_2_to_1(2)/1 -> Bit_1/2
  Bit_Multiplexer_2_to_1(3)/1 -> Bit_1/3
  Bit_Multiplexer_2_to_1(0)/1 -> Bit_0/1
  Clock/1 -> Bit_Multiplexer_2_to_1(8)/2, Bit_Multiplexer_2_to_1(5)/2, Bit_Multiplexer_2_to_1(2)/2, Bit_0/2
  Delay8/1 -> Bit_Comparator(0)/1, Addr_0(1b)/1
  Delay4/1 -> Bit_Comparator(1)/1, Addr_1(1b)/1
  Delay5/1 -> Bit_Comparator(2)/1, Addr_2(1b)/1
  Delay6/1 -> Bit_Comparator(3)/2, Addr_3(1b)/1

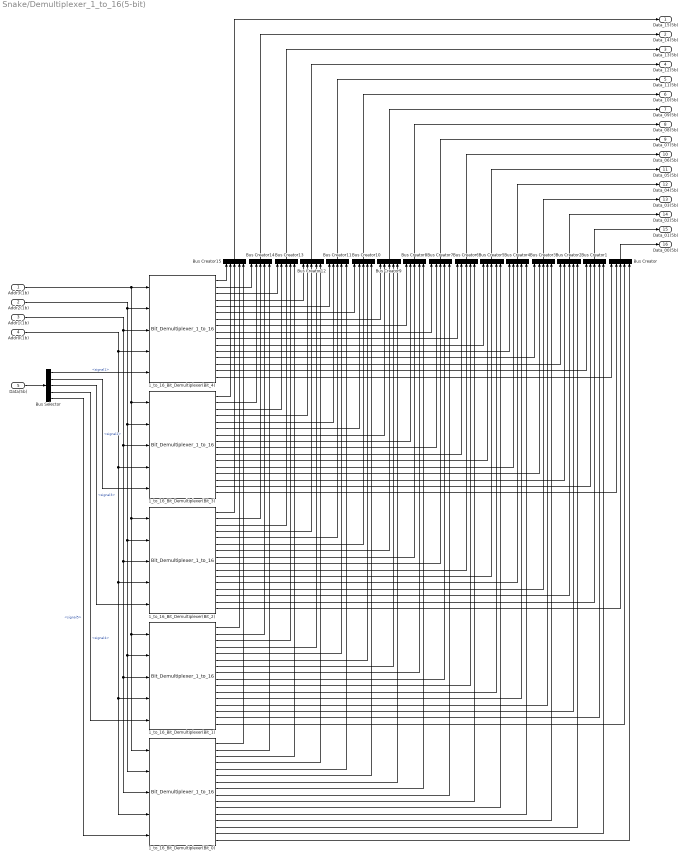
== system Snake/Demultiplexer_1_to_16(5-bit) ==
  Addr3(1b) : Inport
  Addr2(1b) : Inport  Port=2
  Addr1(1b) : Inport  Port=3
  Addr0(1b) : Inport  Port=4
  Data(5b) : Inport  Port=5
  1_to_16_Bit_Demultiplexer(Bit_0) : Bit_Demultiplexers_Lib/Bit_Demultiplexers_Lib/Bit_Demultiplexer_1_to_16
  1_to_16_Bit_Demultiplexer(Bit_1) : Bit_Demultiplexers_Lib/Bit_Demultiplexers_Lib/Bit_Demultiplexer_1_to_16
  1_to_16_Bit_Demultiplexer(Bit_2) : Bit_Demultiplexers_Lib/Bit_Demultiplexers_Lib/Bit_Demultiplexer_1_to_16
  1_to_16_Bit_Demultiplexer(Bit_3) : Bit_Demultiplexers_Lib/Bit_Demultiplexers_Lib/Bit_Demultiplexer_1_to_16
  1_to_16_Bit_Demultiplexer(Bit_4) : Bit_Demultiplexers_Lib/Bit_Demultiplexers_Lib/Bit_Demultiplexer_1_to_16
  Bus Creator{,1..15} (16 alike) : BusCreator  Inputs=5
  Bus Selector : BusSelector  OutputSignals=signal1,signal2,signal3,signal4,signal5
  Data_15(5b) : Outport
  Data_14(5b) : Outport  Port=2
  Data_13(5b) : Outport  Port=3
  Data_12(5b) : Outport  Port=4
  Data_11(5b) : Outport  Port=5
  Data_10(5b) : Outport  Port=6
  Data_09(5b) : Outport  Port=7
  Data_08(5b) : Outport  Port=8
  Data_07(5b) : Outport  Port=9
  Data_06(5b) : Outport  Port=10
  Data_05(5b) : Outport  Port=11
  Data_04(5b) : Outport  Port=12
  Data_03(5b) : Outport  Port=13
  Data_02(5b) : Outport  Port=14
  Data_01(5b) : Outport  Port=15
  Data_00(5b) : Outport  Port=16
  wires:
  Bus Selector/4 -> 1_to_16_Bit_Demultiplexer(Bit_1)/5  "<signal4>"
  Bus Selector/5 -> 1_to_16_Bit_Demultiplexer(Bit_0)/5  "<signal5>"
  Bus Selector/3 -> 1_to_16_Bit_Demultiplexer(Bit_2)/5  "<signal3>"
  Bus Selector/2 -> 1_to_16_Bit_Demultiplexer(Bit_3)/5  "<signal2>"
  Bus Selector/1 -> 1_to_16_Bit_Demultiplexer(Bit_4)/5  "<signal1>"
  Bus Creator15/1 -> Data_15(5b)/1
  Bus Creator14/1 -> Data_14(5b)/1
  Bus Creator13/1 -> Data_13(5b)/1
  Bus Creator12/1 -> Data_12(5b)/1
  Bus Creator11/1 -> Data_11(5b)/1
  Bus Creator10/1 -> Data_10(5b)/1
  Bus Creator9/1 -> Data_09(5b)/1
  Bus Creator8/1 -> Data_08(5b)/1
  Bus Creator7/1 -> Data_07(5b)/1
  Bus Creator6/1 -> Data_06(5b)/1
  Bus Creator5/1 -> Data_05(5b)/1
  Bus Creator4/1 -> Data_04(5b)/1
  Bus Creator3/1 -> Data_03(5b)/1
  Bus Creator2/1 -> Data_02(5b)/1
  Bus Creator1/1 -> Data_01(5b)/1
  Bus Creator/1 -> Data_00(5b)/1
  1_to_16_Bit_Demultiplexer(Bit_0)/16 -> Bus Creator/5
  1_to_16_Bit_Demultiplexer(Bit_0)/15 -> Bus Creator1/5
  1_to_16_Bit_Demultiplexer(Bit_0)/14 -> Bus Creator2/5
  1_to_16_Bit_Demultiplexer(Bit_0)/13 -> Bus Creator3/5
  1_to_16_Bit_Demultiplexer(Bit_0)/12 -> Bus Creator4/5
  1_to_16_Bit_Demultiplexer(Bit_0)/11 -> Bus Creator5/5
  1_to_16_Bit_Demultiplexer(Bit_0)/10 -> Bus Creator6/5
  1_to_16_Bit_Demultiplexer(Bit_0)/9 -> Bus Creator7/5
  1_to_16_Bit_Demultiplexer(Bit_0)/8 -> Bus Creator8/5
  1_to_16_Bit_Demultiplexer(Bit_0)/7 -> Bus Creator9/5
  1_to_16_Bit_Demultiplexer(Bit_0)/6 -> Bus Creator10/5
  1_to_16_Bit_Demultiplexer(Bit_0)/5 -> Bus Creator11/5
  1_to_16_Bit_Demultiplexer(Bit_0)/4 -> Bus Creator12/5
  1_to_16_Bit_Demultiplexer(Bit_0)/3 -> Bus Creator13/5
  1_to_16_Bit_Demultiplexer(Bit_0)/2 -> Bus Creator14/5
  1_to_16_Bit_Demultiplexer(Bit_0)/1 -> Bus Creator15/5
  1_to_16_Bit_Demultiplexer(Bit_1)/16 -> Bus Creator/4
  1_to_16_Bit_Demultiplexer(Bit_1)/15 -> Bus Creator1/4
  1_to_16_Bit_Demultiplexer(Bit_1)/14 -> Bus Creator2/4
  1_to_16_Bit_Demultiplexer(Bit_1)/13 -> Bus Creator3/4
  1_to_16_Bit_Demultiplexer(Bit_1)/12 -> Bus Creator4/4
  1_to_16_Bit_Demultiplexer(Bit_1)/11 -> Bus Creator5/4
  1_to_16_Bit_Demultiplexer(Bit_1)/10 -> Bus Creator6/4
  1_to_16_Bit_Demultiplexer(Bit_1)/9 -> Bus Creator7/4
  1_to_16_Bit_Demultiplexer(Bit_1)/8 -> Bus Creator8/4
  1_to_16_Bit_Demultiplexer(Bit_1)/7 -> Bus Creator9/4
  1_to_16_Bit_Demultiplexer(Bit_1)/6 -> Bus Creator10/4
  1_to_16_Bit_Demultiplexer(Bit_1)/5 -> Bus Creator11/4
  1_to_16_Bit_Demultiplexer(Bit_1)/4 -> Bus Creator12/4
  1_to_16_Bit_Demultiplexer(Bit_1)/3 -> Bus Creator13/4
  1_to_16_Bit_Demultiplexer(Bit_1)/2 -> Bus Creator14/4
  1_to_16_Bit_Demultiplexer(Bit_1)/1 -> Bus Creator15/4
  1_to_16_Bit_Demultiplexer(Bit_2)/16 -> Bus Creator/3
  1_to_16_Bit_Demultiplexer(Bit_2)/15 -> Bus Creator1/3
  1_to_16_Bit_Demultiplexer(Bit_2)/14 -> Bus Creator2/3
  1_to_16_Bit_Demultiplexer(Bit_2)/13 -> Bus Creator3/3
  1_to_16_Bit_Demultiplexer(Bit_2)/12 -> Bus Creator4/3
  1_to_16_Bit_Demultiplexer(Bit_2)/11 -> Bus Creator5/3
  1_to_16_Bit_Demultiplexer(Bit_2)/10 -> Bus Creator6/3
  1_to_16_Bit_Demultiplexer(Bit_2)/9 -> Bus Creator7/3
  1_to_16_Bit_Demultiplexer(Bit_2)/8 -> Bus Creator8/3
  1_to_16_Bit_Demultiplexer(Bit_2)/7 -> Bus Creator9/3
  1_to_16_Bit_Demultiplexer(Bit_2)/6 -> Bus Creator10/3
  1_to_16_Bit_Demultiplexer(Bit_2)/5 -> Bus Creator11/3
  1_to_16_Bit_Demultiplexer(Bit_2)/4 -> Bus Creator12/3
  1_to_16_Bit_Demultiplexer(Bit_2)/3 -> Bus Creator13/3
  1_to_16_Bit_Demultiplexer(Bit_2)/2 -> Bus Creator14/3
  1_to_16_Bit_Demultiplexer(Bit_2)/1 -> Bus Creator15/3
  1_to_16_Bit_Demultiplexer(Bit_3)/16 -> Bus Creator/2
  1_to_16_Bit_Demultiplexer(Bit_3)/15 -> Bus Creator1/2
  1_to_16_Bit_Demultiplexer(Bit_3)/14 -> Bus Creator2/2
  1_to_16_Bit_Demultiplexer(Bit_3)/13 -> Bus Creator3/2
  1_to_16_Bit_Demultiplexer(Bit_3)/12 -> Bus Creator4/2
  1_to_16_Bit_Demultiplexer(Bit_3)/11 -> Bus Creator5/2
  1_to_16_Bit_Demultiplexer(Bit_3)/10 -> Bus Creator6/2
  1_to_16_Bit_Demultiplexer(Bit_3)/9 -> Bus Creator7/2
  1_to_16_Bit_Demultiplexer(Bit_3)/8 -> Bus Creator8/2
  1_to_16_Bit_Demultiplexer(Bit_3)/7 -> Bus Creator9/2
  1_to_16_Bit_Demultiplexer(Bit_3)/6 -> Bus Creator10/2
  1_to_16_Bit_Demultiplexer(Bit_3)/5 -> Bus Creator11/2
  1_to_16_Bit_Demultiplexer(Bit_3)/4 -> Bus Creator12/2
  1_to_16_Bit_Demultiplexer(Bit_3)/3 -> Bus Creator13/2
  1_to_16_Bit_Demultiplexer(Bit_3)/2 -> Bus Creator14/2
  1_to_16_Bit_Demultiplexer(Bit_3)/1 -> Bus Creator15/2
  1_to_16_Bit_Demultiplexer(Bit_4)/16 -> Bus Creator/1
  1_to_16_Bit_Demultiplexer(Bit_4)/15 -> Bus Creator1/1
  1_to_16_Bit_Demultiplexer(Bit_4)/14 -> Bus Creator2/1
  1_to_16_Bit_Demultiplexer(Bit_4)/13 -> Bus Creator3/1
  1_to_16_Bit_Demultiplexer(Bit_4)/12 -> Bus Creator4/1
  1_to_16_Bit_Demultiplexer(Bit_4)/11 -> Bus Creator5/1
  1_to_16_Bit_Demultiplexer(Bit_4)/10 -> Bus Creator6/1
  1_to_16_Bit_Demultiplexer(Bit_4)/9 -> Bus Creator7/1
  1_to_16_Bit_Demultiplexer(Bit_4)/8 -> Bus Creator8/1
  1_to_16_Bit_Demultiplexer(Bit_4)/7 -> Bus Creator9/1
  1_to_16_Bit_Demultiplexer(Bit_4)/6 -> Bus Creator10/1
  1_to_16_Bit_Demultiplexer(Bit_4)/5 -> Bus Creator11/1
  1_to_16_Bit_Demultiplexer(Bit_4)/4 -> Bus Creator12/1
  1_to_16_Bit_Demultiplexer(Bit_4)/3 -> Bus Creator13/1
  1_to_16_Bit_Demultiplexer(Bit_4)/2 -> Bus Creator14/1
  1_to_16_Bit_Demultiplexer(Bit_4)/1 -> Bus Creator15/1
  Data(5b)/1 -> Bus Selector/1
  Addr3(1b)/1 -> 1_to_16_Bit_Demultiplexer(Bit_4)/1, 1_to_16_Bit_Demultiplexer(Bit_3)/1, 1_to_16_Bit_Demultiplexer(Bit_2)/1, 1_to_16_Bit_Demultiplexer(Bit_1)/1, 1_to_16_Bit_Demultiplexer(Bit_0)/1
  Addr2(1b)/1 -> 1_to_16_Bit_Demultiplexer(Bit_3)/2, 1_to_16_Bit_Demultiplexer(Bit_2)/2, 1_to_16_Bit_Demultiplexer(Bit_1)/2, 1_to_16_Bit_Demultiplexer(Bit_0)/2, 1_to_16_Bit_Demultiplexer(Bit_4)/2
  Addr1(1b)/1 -> 1_to_16_Bit_Demultiplexer(Bit_3)/3, 1_to_16_Bit_Demultiplexer(Bit_2)/3, 1_to_16_Bit_Demultiplexer(Bit_1)/3, 1_to_16_Bit_Demultiplexer(Bit_0)/3, 1_to_16_Bit_Demultiplexer(Bit_4)/3
  Addr0(1b)/1 -> 1_to_16_Bit_Demultiplexer(Bit_3)/4, 1_to_16_Bit_Demultiplexer(Bit_2)/4, 1_to_16_Bit_Demultiplexer(Bit_1)/4, 1_to_16_Bit_Demultiplexer(Bit_0)/4, 1_to_16_Bit_Demultiplexer(Bit_4)/4
